simulink model "udp_with_svm"  (R2023b)
settings: Solver=VariableStepAuto  StartTime=0.0  StopTime=inf  RelTol=1e-3
libraries: alterasoclib x1
settings Model: Creator=user  LastModifiedBy=user
settings OptimizationCC: BlockReduction=off  ConditionallyExecuteInputs=off  DefaultParameterBehavior=Inlined
settings DebuggingCC: AlgebraicLoopMsg=error  ParameterOverflowMsg=none
settings HardwareCC: ProdBitPerPointer=32  ProdBitPerSizeT=32  ProdBitPerPtrDiffT=32  ProdLargestAtomicFloat=None  ProdIntDivRoundTo=Undefined  ProdEndianess=Unspecified  ProdWordSize=32  ProdHWDeviceType=ASIC/FPGA->ASIC/FPGA  TargetBitPerPointer=64  TargetBitPerSizeT=64  TargetBitPerPtrDiffT=64  TargetLongLongMode=on  TargetIntDivRoundTo=Zero  TargetEndianess=LittleEndian  TargetWordSize=64  TargetHWDeviceType=Custom Processor->MATLAB Host Computer  ProdEqTarget=off

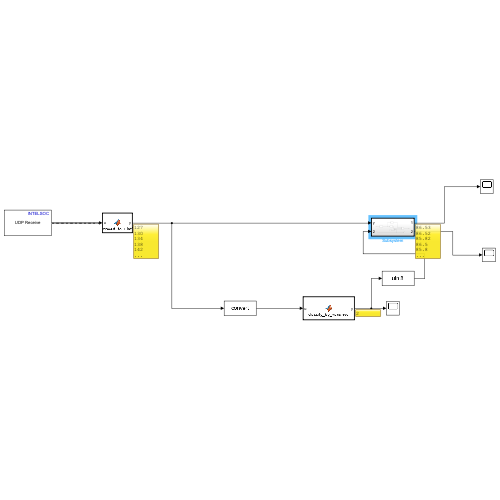
[thumbnail: Simulink's stored preview of the top-level diagram]
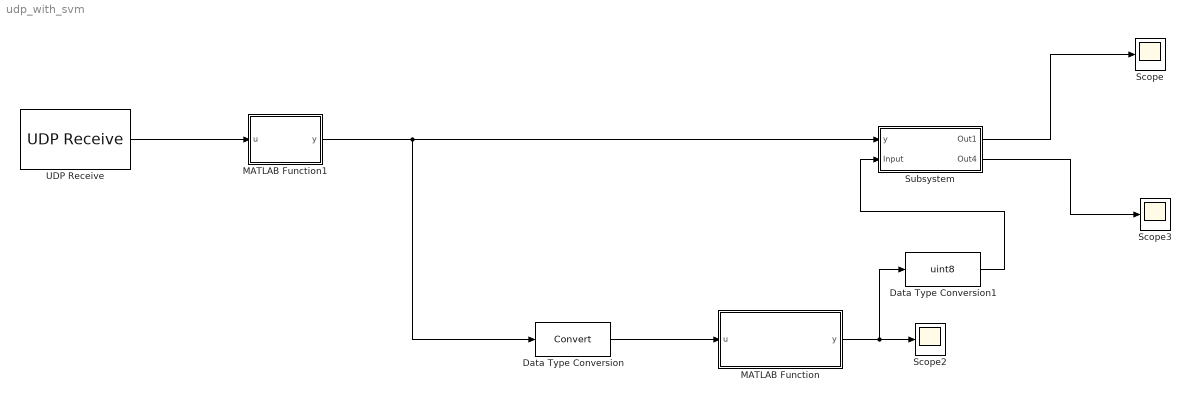
== system udp_with_svm ==
  Data Type Conversion : DataTypeConversion  SaturateOnIntegerOverflow=off  RndMeth=Floor
  Data Type Conversion1 : DataTypeConversion  OutDataTypeStr=uint8  SaturateOnIntegerOverflow=off  RndMeth=Floor
  MATLAB Function : MATLAB Function  TreatAsAtomicUnit=on
  MATLAB Function1 : MATLAB Function  TreatAsAtomicUnit=on
  Scope : Scope
  Scope2 : Scope
  Scope3 : Scope
  Subsystem : Subsystem  TreatAsAtomicUnit=on
  UDP Receive : alterasoclib/UDP Receive  localURL='0.0.0.0'  localPort=25000  remoteURL='0.0.0.0'  remotePort=-1  recvBufferSize=8192  dims=255  signalDatatype=uint8  isVarSize=on  showBlockingTime=on  blockingTime=inf  sampletime=0.01  blockPlatform=INTELSOC
  wires:
  Data Type Conversion/1 -> MATLAB Function/1(u)
  MATLAB Function/1(y) -> Data Type Conversion1/1, Scope2/1
  Subsystem/1(Out1) -> Scope/1
  Data Type Conversion1/1 -> Subsystem/2(Input)
  Subsystem/2(Out4) -> Scope3/1
  MATLAB Function1/1(y) -> Data Type Conversion/1, Subsystem/1(y)
  UDP Receive/1 -> MATLAB Function1/1(u)

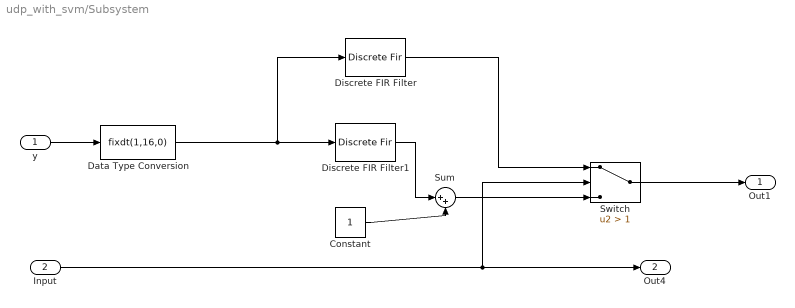
== system udp_with_svm/Subsystem ==
  y : Inport  OutDataTypeStr=uint8
  Input : Inport  Port=2
  Constant : Constant
  Data Type Conversion : DataTypeConversion  OutDataTypeStr=fixdt(1,16,0)  SaturateOnIntegerOverflow=off  RndMeth=Floor
  Discrete FIR Filter : DiscreteFir
  Discrete FIR Filter1 : DiscreteFir
  Sum : Sum  Inputs=|++  OutDataTypeStr=uint8
  Switch : Switch  Criteria=u2 > Threshold  Threshold=1  SaturateOnIntegerOverflow=off  InputSameDT=off
  Out1 : Outport
  Out4 : Outport  Port=2  VectorParamsAs1DForOutWhenUnconnected=off
  wires:
  y/1 -> Data Type Conversion/1
  Input/1 -> Switch/2, Out4/1
  Switch/1 -> Out1/1
  Data Type Conversion/1 -> Discrete FIR Filter/1, Discrete FIR Filter1/1
  Discrete FIR Filter/1 -> Switch/1
  Constant/1 -> Sum/2
  Discrete FIR Filter1/1 -> Sum/1
  Sum/1 -> Switch/3

== matlab function udp_with_svm/MATLAB Function ==
  data: u input; y output
function y = classify_by_variance(u)
% Classifies a 256x1 input vector based on its variance.

% Input:
%   u: A 256x1 double vector representing the input signal (values 0-255).

% Output:
%   y: A scalar double value, either 1 or 2, representing the class label.

% Calculate the variance of the input vector:
variance_u = var(u);

% Define a threshold for "high" variance (adjust as needed):
% IMPORTANT: Tune this threshold based on your data!
% The range 0-255 suggests a lower threshold than my previous example.
% Start by analyzing the variance of your data in MATLAB to get a good range.
variance_threshold = 1000;  % Example, tune this!  Start lower, e.g. 100, then adjust

% Classify based on the variance:
if variance_u < variance_threshold
    y = 1;  % Low variance, class 1
else
    y = 2;  % High variance, class 2
end


end

== matlab function udp_with_svm/MATLAB Function1 ==
  data: u input; y output
function y = convert_to_uint8(u)
    persistent buffer count last_valid_output;
    
    if isempty(buffer)
        buffer = zeros(1, 400, 'uint8'); 
        count = 0; 
        last_valid_output = zeros(1, 400, 'uint8'); 
    end
    

    count = count + 1;
    buffer(mod(count-1, 400) + 1) = uint8(u);  

    if count >= 400
        last_valid_output = buffer;  
        count = 0;  
    end
    
    y = last_valid_output;
end
